simulink model "Blupanda"  (R2023a)
settings: Solver=VariableStepAuto  StartTime=0.0  StopTime=10.0  RelTol=1e-3
(part 2 of 2)

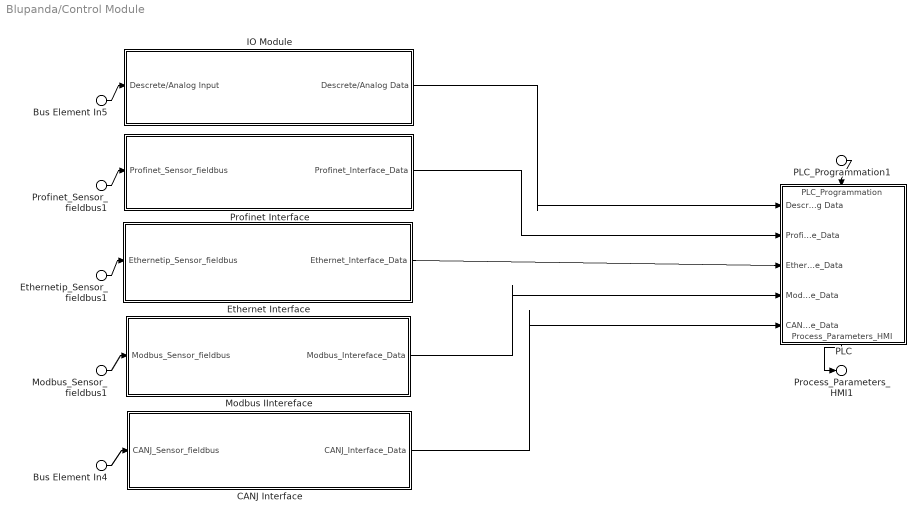
== system Blupanda/Control Module ==
  PLC_Programmation1 : Inport  PortName=PLC_Programmation
  Profinet_Sensor_fieldbus1 : Inport  Port=2  PortName=Profinet_Sensor_fieldbus
  Ethernetip_Sensor_fieldbus1 : Inport  Port=3  PortName=Ethernetip_Sensor_fieldbus
  Bus Element In4 : Inport  Port=4  PortName=CANJ_Sensor_fieldbus
  Bus Element In5 : Inport  Port=5  PortName=Descrete/Analog Input
  Modbus_Sensor_fieldbus1 : Inport  Port=6  PortName=Modbus_Sensor_fieldbus
  CANJ Interface : Subsystem
      settings: PortSchema="{\"entries\":[{\"content\":{\"headerSize\":26,\"margin\":15,\"minimumSpacing\":25,\"sides\":[{\"content\":{\"connectorIds\":[\"In1\"]},\"type\":\"ConnectorPlacement.EquallySpacedRectSide\",\"uuid\":\"ff8f3bf2-d6f6-4ecc-9677-a0e5f5ade440\"},{\"content\":{\"connectorIds\":[\"Out1\"],\"side\":\"RIGHT\"},\"type\":\"ConnectorPlacement.EquallySpacedRectSide\",\"uuid\":\"fe155757-f3d5-40d8-a583-dbbc24843437\"},{\"content\":{\"side\":\"TOP\"},\"type\":\"ConnectorPlacement.EquallySpacedRectSide\",\"uuid\":\"51bc4fd0-0675-45de-93bd-0dc8d94c5489\"}]},\"type\":\"ConnectorPlacement.EquallySpacedConnector\",\"uuid\":\"7eb8fdf8-dbe2-49f3-b9bd-384f85dcc997\"}],\"packageUris\":[\"http://schema.mathworks.com/mf0/Connector/R2020b\"],\"version\":\"1.0\"}"
  Ethernet Interface : Subsystem
      settings: PortSchema="{\"entries\":[{\"content\":{\"headerSize\":26,\"margin\":15,\"minimumSpacing\":25,\"sides\":[{\"content\":{\"connectorIds\":[\"In1\"]},\"type\":\"ConnectorPlacement.EquallySpacedRectSide\",\"uuid\":\"ff8f3bf2-d6f6-4ecc-9677-a0e5f5ade440\"},{\"content\":{\"connectorIds\":[\"Out1\"],\"side\":\"RIGHT\"},\"type\":\"ConnectorPlacement.EquallySpacedRectSide\",\"uuid\":\"fe155757-f3d5-40d8-a583-dbbc24843437\"},{\"content\":{\"side\":\"TOP\"},\"type\":\"ConnectorPlacement.EquallySpacedRectSide\",\"uuid\":\"51bc4fd0-0675-45de-93bd-0dc8d94c5489\"}]},\"type\":\"ConnectorPlacement.EquallySpacedConnector\",\"uuid\":\"7eb8fdf8-dbe2-49f3-b9bd-384f85dcc997\"}],\"packageUris\":[\"http://schema.mathworks.com/mf0/Connector/R2020b\"],\"version\":\"1.0\"}"
  IO Module : Subsystem
      settings: PortSchema="{\"entries\":[{\"content\":{\"headerSize\":26,\"margin\":15,\"minimumSpacing\":25,\"sides\":[{\"content\":{\"connectorIds\":[\"In1\"]},\"type\":\"ConnectorPlacement.EquallySpacedRectSide\",\"uuid\":\"ff8f3bf2-d6f6-4ecc-9677-a0e5f5ade440\"},{\"content\":{\"connectorIds\":[\"Out1\"],\"side\":\"RIGHT\"},\"type\":\"ConnectorPlacement.EquallySpacedRectSide\",\"uuid\":\"fe155757-f3d5-40d8-a583-dbbc24843437\"},{\"content\":{\"side\":\"TOP\"},\"type\":\"ConnectorPlacement.EquallySpacedRectSide\",\"uuid\":\"51bc4fd0-0675-45de-93bd-0dc8d94c5489\"}]},\"type\":\"ConnectorPlacement.EquallySpacedConnector\",\"uuid\":\"7eb8fdf8-dbe2-49f3-b9bd-384f85dcc997\"}],\"packageUris\":[\"http://schema.mathworks.com/mf0/Connector/R2020b\"],\"version\":\"1.0\"}"
  Modbus IIntereface : Subsystem
      settings: PortSchema="{\"entries\":[{\"content\":{\"headerSize\":26,\"margin\":15,\"minimumSpacing\":25,\"sides\":[{\"content\":{\"connectorIds\":[\"In1\"]},\"type\":\"ConnectorPlacement.EquallySpacedRectSide\",\"uuid\":\"ff8f3bf2-d6f6-4ecc-9677-a0e5f5ade440\"},{\"content\":{\"connectorIds\":[\"Out1\"],\"side\":\"RIGHT\"},\"type\":\"ConnectorPlacement.EquallySpacedRectSide\",\"uuid\":\"fe155757-f3d5-40d8-a583-dbbc24843437\"},{\"content\":{\"side\":\"TOP\"},\"type\":\"ConnectorPlacement.EquallySpacedRectSide\",\"uuid\":\"51bc4fd0-0675-45de-93bd-0dc8d94c5489\"}]},\"type\":\"ConnectorPlacement.EquallySpacedConnector\",\"uuid\":\"7eb8fdf8-dbe2-49f3-b9bd-384f85dcc997\"}],\"packageUris\":[\"http://schema.mathworks.com/mf0/Connector/R2020b\"],\"version\":\"1.0\"}"
  PLC : Subsystem
      settings: PortSchema="{\"entries\":[{\"content\":{\"headerSize\":26,\"margin\":15,\"minimumSpacing\":25,\"sides\":[{\"content\":{\"connectorIds\":[\"In1\",\"In4\",\"In5\",\"In6\",\"In2\"]},\"type\":\"ConnectorPlacement.EquallySpacedRectSide\",\"uuid\":\"ff8f3bf2-d6f6-4ecc-9677-a0e5f5ade440\"},{\"content\":{\"side\":\"RIGHT\"},\"type\":\"ConnectorPlacement.EquallySpacedRectSide\",\"uuid\":\"fe155757-f3d5-40d8-a583-dbbc24843437\"},{\"content\":{\"connectorIds\":[\"In3\"],\"side\":\"TOP\"},\"type\":\"ConnectorPlacement.EquallySpacedRectSide\",\"uuid\":\"51bc4fd0-0675-45de-93bd-0dc8d94c5489\"},{\"content\":{\"connectorIds\":[\"Out1\"],\"side\":\"BOTTOM\"},\"type\":\"ConnectorPlacement.EquallySpacedRectSide\",\"uuid\":\"b7b44f41-0e2c-4bbd-9aa1-2b70573de7d3\"}]},\"type\":\"ConnectorPlacement.EquallySpacedConnector\",\"uuid\":\"7eb8fdf8-dbe2-49f3-b9bd-384f85dcc997\"}],\"packageUris\":[\"http://schema.mathworks.com/mf0/Connector/R2020b\"],\"version\":\"1.0\"}"
  Profinet Interface : Subsystem
      settings: PortSchema="{\"entries\":[{\"content\":{\"headerSize\":26,\"margin\":15,\"minimumSpacing\":25,\"sides\":[{\"content\":{\"connectorIds\":[\"In1\"]},\"type\":\"ConnectorPlacement.EquallySpacedRectSide\",\"uuid\":\"ff8f3bf2-d6f6-4ecc-9677-a0e5f5ade440\"},{\"content\":{\"connectorIds\":[\"Out1\"],\"side\":\"RIGHT\"},\"type\":\"ConnectorPlacement.EquallySpacedRectSide\",\"uuid\":\"fe155757-f3d5-40d8-a583-dbbc24843437\"},{\"content\":{\"side\":\"TOP\"},\"type\":\"ConnectorPlacement.EquallySpacedRectSide\",\"uuid\":\"51bc4fd0-0675-45de-93bd-0dc8d94c5489\"}]},\"type\":\"ConnectorPlacement.EquallySpacedConnector\",\"uuid\":\"7eb8fdf8-dbe2-49f3-b9bd-384f85dcc997\"}],\"packageUris\":[\"http://schema.mathworks.com/mf0/Connector/R2020b\"],\"version\":\"1.0\"}"
  Process_Parameters_HMI1 : Outport  PortName=Process_Parameters_HMI
  wires:
  Modbus_Sensor_fieldbus1/1 -> Modbus IIntereface/1(Modbus_Sensor_fieldbus)
  Profinet_Sensor_fieldbus1/1 -> Profinet Interface/1(Profinet_Sensor_fieldbus)
  Ethernetip_Sensor_fieldbus1/1 -> Ethernet Interface/1(Ethernetip_Sensor_fieldbus)
  Profinet Interface/1(Profinet_Interface_Data) -> PLC/4(Profinet_Interface_Data)
  Modbus IIntereface/1(Modbus_Intereface_Data) -> PLC/6(Modbus_Intereface_Data)
  PLC/1(Process_Parameters_HMI) -> Process_Parameters_HMI1/1
  Ethernet Interface/1(Ethernet_Interface_Data) -> PLC/5(Ethernet_Interface_Data)
  PLC_Programmation1/1 -> PLC/3(PLC_Programmation)
  CANJ Interface/1(CANJ_Interface_Data) -> PLC/2(CANJ_Interface_Data)
  Bus Element In4/1 -> CANJ Interface/1(CANJ_Sensor_fieldbus)
  IO Module/1(Descrete/Analog Data) -> PLC/1(Descrete/Analog Data)
  Bus Element In5/1 -> IO Module/1(Descrete/Analog Input)

== system Blupanda/Deutsch 6-pin Connector ==
  Bus Element In1 : Inport  PortName=XGCS460B201_CANJ_Data
  Bus Element Out1 : Outport  PortName=CANJ_Sensor_fieldbus

== system Blupanda/EthernetIP_network ==
  Bus Element In1 : Inport  PortName=ethernet ip data
  Bus Element Out1 : Outport  PortName=Ethernetip_Sensor_fieldbus

== system Blupanda/HMI ==
  Bus Element In1 : Inport  PortName=Process_Parameters_HMI

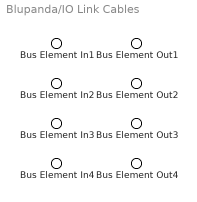
== system Blupanda/IO Link Cables ==
  Bus Element In1 : Inport  PortName=XGCS 89 01201_IOLimk_data
  Bus Element In2 : Inport  Port=2  PortName=XGCS 49 01201_IOLink_data
  Bus Element In3 : Inport  Port=3  PortName=M18_IOLink_data
  Bus Element In4 : Inport  Port=4  PortName=M30_IOLink_data
  Bus Element Out1 : Outport  PortName=XGCS 89 01201_IOLimk_data_2_master
  Bus Element Out2 : Outport  Port=2  PortName=XGCS 49 01201_IOLink_data_2_master
  Bus Element Out3 : Outport  Port=3  PortName=M18_IOLink_data_2_master
  Bus Element Out4 : Outport  Port=4  PortName=M30_IOLink_data_2_masters

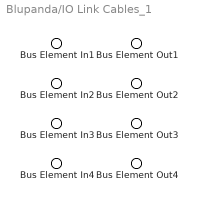
== system Blupanda/IO Link Cables_1 ==
  Bus Element In1 : Inport  PortName=XGCS 89 01201_IOLimk_data
  Bus Element In2 : Inport  Port=2  PortName=XGCS 49 01201_IOLink_data
  Bus Element In3 : Inport  Port=3  PortName=M18_IOLink_data
  Bus Element In4 : Inport  Port=4  PortName=M30_IOLink_data
  Bus Element Out1 : Outport  PortName=XGCS 89 01201_IOLimk_data_2_master
  Bus Element Out2 : Outport  Port=2  PortName=XGCS 49 01201_IOLink_data_2_master
  Bus Element Out3 : Outport  Port=3  PortName=M18_IOLink_data_2_master
  Bus Element Out4 : Outport  Port=4  PortName=M30_IOLink_data_2_masters

== system Blupanda/IOLink_master_EthernetIP ==
  Bus Element In1 : Inport  PortName=XGCS 49 01201_IOLink_data
  Bus Element In2 : Inport  Port=2  PortName=XGCS 89 01201_IOLimk_data
  Bus Element In3 : Inport  Port=3  PortName=M18_IOLink_data
  Bus Element In4 : Inport  Port=4  PortName=M30_IOLink_data
  Bus Element Out1 : Outport  PortName=IOLink_master_Profinet_serial_data_EthernetIP

== system Blupanda/IOLink_master_Profinet ==
  Bus Element In1 : Inport  PortName=XGCS 89 01201_IOLimk_data_2_master
  Bus Element In2 : Inport  Port=2  PortName=XGCS 49 01201_IOLink_data_2_master
  Bus Element In3 : Inport  Port=3  PortName=M18_IOLink_data_2_master
  Bus Element In4 : Inport  Port=4  PortName=M30_IOLink_data_2_masters
  Bus Element Out1 : Outport  PortName=IOLink_master_Profinet_serial_data_profinet

== system Blupanda/Interface_box_network_1 ==
  Bus Element In1 : Inport  PortName="XGSZ84 PNT  _serial_data_Profinet"
  Bus Element Out1 : Outport  PortName="XGSZ84 PNT  _serial_data_Profinet_2_network"

== system Blupanda/Interface_box_network_2 ==
  Bus Element In1 : Inport  PortName=XGSZ 84 EIP _serial_data_ethernet
  Bus Element Out1 : Outport  PortName=XGSZ 84 EIP _serial_data_ethernet_2_network

== system Blupanda/Interface_box_network_3 ==
  Bus Element In1 : Inport  PortName=XGSZ84 ETH _serial_data_Mobdus
  Bus Element Out1 : Outport  PortName=XGSZ84 ETH _serial_data_Mobdus_2_network

== system Blupanda/M12 to Ethernet 0 ==
  Bus Element In1 : Inport  PortName=XGCS 850C 201_ModusTCp_Data
  Bus Element Out1 : Outport  PortName=""

== system Blupanda/M12 to Ethernet 1 ==
  Bus Element In1 : Inport  PortName=XGCS 850C 201_Ethernetp_Data
  Bus Element Out1 : Outport  PortName=XGCS 850C 201_Ethernetp_Data_2_swtich

== system Blupanda/M12 to Ethernet 2 ==
  Bus Element In1 : Inport  PortName=XGCS 850C 201_Profinet_Data
  Bus Element Out1 : Outport  PortName=XGCS 850C 201_Profinet_Data_2_network

== system Blupanda/ModbusTCP_Network ==
  Bus Element In1 : Inport  PortName=XGSZ84 ETH _serial_data_Mobdus_2_network
  Bus Element In2 : Inport  Port=2  PortName=XGCS 850C 201_ModusTCp_Data_2_network
  Bus Element Out1 : Outport  PortName=Modbus_Sensor_fieldbus

== system Blupanda/Profinet_network ==
  Bus Element In2 : Inport  PortName=IOLink_master_Profinet_serial_data_profinet
  Bus Element In1 : Inport  Port=2  PortName="XGSZ84 PNT  _serial_data_Profinet_2_network"
  Bus Element In3 : Inport  Port=3  PortName=XGCS 850C 201_Profinet_Data
  Bus Element Out1 : Outport  PortName=Profinet_Sensor_fieldbus

== system Blupanda/RFID_CANJ ==
  XGCS460B201 : Subsystem
      settings: PortSchema="{\"entries\":[{\"content\":{\"headerSize\":26,\"margin\":15,\"minimumSpacing\":25,\"sides\":[{\"content\":{},\"type\":\"ConnectorPlacement.EquallySpacedRectSide\",\"uuid\":\"ff8f3bf2-d6f6-4ecc-9677-a0e5f5ade440\"},{\"content\":{\"connectorIds\":[\"Out1\"],\"side\":\"RIGHT\"},\"type\":\"ConnectorPlacement.EquallySpacedRectSide\",\"uuid\":\"fe155757-f3d5-40d8-a583-dbbc24843437\"},{\"content\":{\"side\":\"TOP\"},\"type\":\"ConnectorPlacement.EquallySpacedRectSide\",\"uuid\":\"51bc4fd0-0675-45de-93bd-0dc8d94c5489\"}]},\"type\":\"ConnectorPlacement.EquallySpacedConnector\",\"uuid\":\"7eb8fdf8-dbe2-49f3-b9bd-384f85dcc997\"}],\"packageUris\":[\"http://schema.mathworks.com/mf0/Connector/R2020b\"],\"version\":\"1.0\"}"
  XGCS460B202_CANJ_Data1 : Outport  PortName=XGCS460B201_CANJ_Data
  wires:
  XGCS460B201/1(XGCS460B201_CANJ_Data) -> XGCS460B202_CANJ_Data1/1

== system Blupanda/RFID_EthernetIP ==
  "XGCS 850C 201 " : Subsystem
      settings: PortSchema="{\"entries\":[{\"content\":{\"headerSize\":26,\"margin\":15,\"minimumSpacing\":25,\"sides\":[{\"content\":{},\"type\":\"ConnectorPlacement.EquallySpacedRectSide\",\"uuid\":\"ff8f3bf2-d6f6-4ecc-9677-a0e5f5ade440\"},{\"content\":{\"side\":\"RIGHT\"},\"type\":\"ConnectorPlacement.EquallySpacedRectSide\",\"uuid\":\"fe155757-f3d5-40d8-a583-dbbc24843437\"},{\"content\":{\"connectorIds\":[\"Out1\"],\"side\":\"TOP\"},\"type\":\"ConnectorPlacement.EquallySpacedRectSide\",\"uuid\":\"51bc4fd0-0675-45de-93bd-0dc8d94c5489\"},{\"content\":{\"side\":\"BOTTOM\"},\"type\":\"ConnectorPlacement.EquallySpacedRectSide\",\"uuid\":\"69d4bc1c-5af7-467d-9dcb-7dfd5dc85590\"}]},\"type\":\"ConnectorPlacement.EquallySpacedConnector\",\"uuid\":\"7eb8fdf8-dbe2-49f3-b9bd-384f85dcc997\"}],\"packageUris\":[\"http://schema.mathworks.com/mf0/Connector/R2020b\"],\"version\":\"1.0\"}"
  XGCS 850C 201_Ethernetp_Data1 : Outport  PortName=XGCS 850C 201_Ethernetp_Data
  wires:
  "XGCS 850C 201 "/1(XGCS 850C 201_Ethernetp_Data) -> XGCS 850C 201_Ethernetp_Data1/1

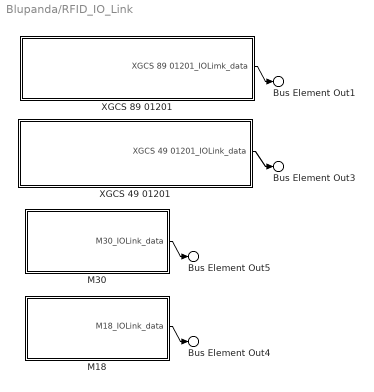
== system Blupanda/RFID_IO_Link ==
  M18 : Subsystem
      settings: PortSchema="{\"entries\":[{\"content\":{\"headerSize\":26,\"margin\":15,\"minimumSpacing\":25,\"sides\":[{\"content\":{},\"type\":\"ConnectorPlacement.EquallySpacedRectSide\",\"uuid\":\"ff8f3bf2-d6f6-4ecc-9677-a0e5f5ade440\"},{\"content\":{\"connectorIds\":[\"Out1\"],\"side\":\"RIGHT\"},\"type\":\"ConnectorPlacement.EquallySpacedRectSide\",\"uuid\":\"fe155757-f3d5-40d8-a583-dbbc24843437\"},{\"content\":{\"side\":\"TOP\"},\"type\":\"ConnectorPlacement.EquallySpacedRectSide\",\"uuid\":\"51bc4fd0-0675-45de-93bd-0dc8d94c5489\"}]},\"type\":\"ConnectorPlacement.EquallySpacedConnector\",\"uuid\":\"7eb8fdf8-dbe2-49f3-b9bd-384f85dcc997\"}],\"packageUris\":[\"http://schema.mathworks.com/mf0/Connector/R2020b\"],\"version\":\"1.0\"}"
  M30 : Subsystem
      settings: PortSchema="{\"entries\":[{\"content\":{\"headerSize\":26,\"margin\":15,\"minimumSpacing\":25,\"sides\":[{\"content\":{},\"type\":\"ConnectorPlacement.EquallySpacedRectSide\",\"uuid\":\"ff8f3bf2-d6f6-4ecc-9677-a0e5f5ade440\"},{\"content\":{\"connectorIds\":[\"Out1\"],\"side\":\"RIGHT\"},\"type\":\"ConnectorPlacement.EquallySpacedRectSide\",\"uuid\":\"fe155757-f3d5-40d8-a583-dbbc24843437\"},{\"content\":{\"side\":\"TOP\"},\"type\":\"ConnectorPlacement.EquallySpacedRectSide\",\"uuid\":\"51bc4fd0-0675-45de-93bd-0dc8d94c5489\"}]},\"type\":\"ConnectorPlacement.EquallySpacedConnector\",\"uuid\":\"7eb8fdf8-dbe2-49f3-b9bd-384f85dcc997\"}],\"packageUris\":[\"http://schema.mathworks.com/mf0/Connector/R2020b\"],\"version\":\"1.0\"}"
  XGCS 49 01201 : Subsystem
      settings: PortSchema="{\"entries\":[{\"content\":{\"headerSize\":26,\"margin\":15,\"minimumSpacing\":25,\"sides\":[{\"content\":{},\"type\":\"ConnectorPlacement.EquallySpacedRectSide\",\"uuid\":\"ff8f3bf2-d6f6-4ecc-9677-a0e5f5ade440\"},{\"content\":{\"connectorIds\":[\"Out1\"],\"side\":\"RIGHT\"},\"type\":\"ConnectorPlacement.EquallySpacedRectSide\",\"uuid\":\"fe155757-f3d5-40d8-a583-dbbc24843437\"},{\"content\":{\"side\":\"TOP\"},\"type\":\"ConnectorPlacement.EquallySpacedRectSide\",\"uuid\":\"51bc4fd0-0675-45de-93bd-0dc8d94c5489\"}]},\"type\":\"ConnectorPlacement.EquallySpacedConnector\",\"uuid\":\"7eb8fdf8-dbe2-49f3-b9bd-384f85dcc997\"}],\"packageUris\":[\"http://schema.mathworks.com/mf0/Connector/R2020b\"],\"version\":\"1.0\"}"
  XGCS 89 01201 : Subsystem
      settings: PortSchema="{\"entries\":[{\"content\":{\"headerSize\":26,\"margin\":15,\"minimumSpacing\":25,\"sides\":[{\"content\":{},\"type\":\"ConnectorPlacement.EquallySpacedRectSide\",\"uuid\":\"ff8f3bf2-d6f6-4ecc-9677-a0e5f5ade440\"},{\"content\":{\"connectorIds\":[\"Out1\"],\"side\":\"RIGHT\"},\"type\":\"ConnectorPlacement.EquallySpacedRectSide\",\"uuid\":\"fe155757-f3d5-40d8-a583-dbbc24843437\"},{\"content\":{\"side\":\"TOP\"},\"type\":\"ConnectorPlacement.EquallySpacedRectSide\",\"uuid\":\"51bc4fd0-0675-45de-93bd-0dc8d94c5489\"}]},\"type\":\"ConnectorPlacement.EquallySpacedConnector\",\"uuid\":\"7eb8fdf8-dbe2-49f3-b9bd-384f85dcc997\"}],\"packageUris\":[\"http://schema.mathworks.com/mf0/Connector/R2020b\"],\"version\":\"1.0\"}"
  Bus Element Out1 : Outport  PortName=XGCS 89 01201_IOLimk_data
  Bus Element Out3 : Outport  Port=2  PortName=XGCS 49 01201_IOLink_data
  Bus Element Out4 : Outport  Port=3  PortName=M18_IOLink_data
  Bus Element Out5 : Outport  Port=4  PortName=M30_IOLink_data
  wires:
  XGCS 89 01201/1(XGCS 89 01201_IOLimk_data) -> Bus Element Out1/1
  XGCS 49 01201/1(XGCS 49 01201_IOLink_data) -> Bus Element Out3/1
  M30/1(M30_IOLink_data) -> Bus Element Out5/1
  M18/1(M18_IOLink_data) -> Bus Element Out4/1

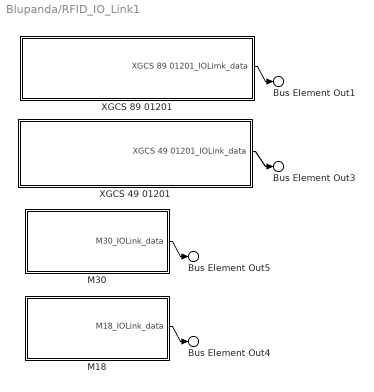
== system Blupanda/RFID_IO_Link1 ==
  M18 : Subsystem
      settings: PortSchema="{\"entries\":[{\"content\":{\"headerSize\":26,\"margin\":15,\"minimumSpacing\":25,\"sides\":[{\"content\":{},\"type\":\"ConnectorPlacement.EquallySpacedRectSide\",\"uuid\":\"ff8f3bf2-d6f6-4ecc-9677-a0e5f5ade440\"},{\"content\":{\"connectorIds\":[\"Out1\"],\"side\":\"RIGHT\"},\"type\":\"ConnectorPlacement.EquallySpacedRectSide\",\"uuid\":\"fe155757-f3d5-40d8-a583-dbbc24843437\"},{\"content\":{\"side\":\"TOP\"},\"type\":\"ConnectorPlacement.EquallySpacedRectSide\",\"uuid\":\"51bc4fd0-0675-45de-93bd-0dc8d94c5489\"}]},\"type\":\"ConnectorPlacement.EquallySpacedConnector\",\"uuid\":\"7eb8fdf8-dbe2-49f3-b9bd-384f85dcc997\"}],\"packageUris\":[\"http://schema.mathworks.com/mf0/Connector/R2020b\"],\"version\":\"1.0\"}"
  M30 : Subsystem
      settings: PortSchema="{\"entries\":[{\"content\":{\"headerSize\":26,\"margin\":15,\"minimumSpacing\":25,\"sides\":[{\"content\":{},\"type\":\"ConnectorPlacement.EquallySpacedRectSide\",\"uuid\":\"ff8f3bf2-d6f6-4ecc-9677-a0e5f5ade440\"},{\"content\":{\"connectorIds\":[\"Out1\"],\"side\":\"RIGHT\"},\"type\":\"ConnectorPlacement.EquallySpacedRectSide\",\"uuid\":\"fe155757-f3d5-40d8-a583-dbbc24843437\"},{\"content\":{\"side\":\"TOP\"},\"type\":\"ConnectorPlacement.EquallySpacedRectSide\",\"uuid\":\"51bc4fd0-0675-45de-93bd-0dc8d94c5489\"}]},\"type\":\"ConnectorPlacement.EquallySpacedConnector\",\"uuid\":\"7eb8fdf8-dbe2-49f3-b9bd-384f85dcc997\"}],\"packageUris\":[\"http://schema.mathworks.com/mf0/Connector/R2020b\"],\"version\":\"1.0\"}"
  XGCS 49 01201 : Subsystem
      settings: PortSchema="{\"entries\":[{\"content\":{\"headerSize\":26,\"margin\":15,\"minimumSpacing\":25,\"sides\":[{\"content\":{},\"type\":\"ConnectorPlacement.EquallySpacedRectSide\",\"uuid\":\"ff8f3bf2-d6f6-4ecc-9677-a0e5f5ade440\"},{\"content\":{\"connectorIds\":[\"Out1\"],\"side\":\"RIGHT\"},\"type\":\"ConnectorPlacement.EquallySpacedRectSide\",\"uuid\":\"fe155757-f3d5-40d8-a583-dbbc24843437\"},{\"content\":{\"side\":\"TOP\"},\"type\":\"ConnectorPlacement.EquallySpacedRectSide\",\"uuid\":\"51bc4fd0-0675-45de-93bd-0dc8d94c5489\"}]},\"type\":\"ConnectorPlacement.EquallySpacedConnector\",\"uuid\":\"7eb8fdf8-dbe2-49f3-b9bd-384f85dcc997\"}],\"packageUris\":[\"http://schema.mathworks.com/mf0/Connector/R2020b\"],\"version\":\"1.0\"}"
  XGCS 89 01201 : Subsystem
      settings: PortSchema="{\"entries\":[{\"content\":{\"headerSize\":26,\"margin\":15,\"minimumSpacing\":25,\"sides\":[{\"content\":{},\"type\":\"ConnectorPlacement.EquallySpacedRectSide\",\"uuid\":\"ff8f3bf2-d6f6-4ecc-9677-a0e5f5ade440\"},{\"content\":{\"connectorIds\":[\"Out1\"],\"side\":\"RIGHT\"},\"type\":\"ConnectorPlacement.EquallySpacedRectSide\",\"uuid\":\"fe155757-f3d5-40d8-a583-dbbc24843437\"},{\"content\":{\"side\":\"TOP\"},\"type\":\"ConnectorPlacement.EquallySpacedRectSide\",\"uuid\":\"51bc4fd0-0675-45de-93bd-0dc8d94c5489\"}]},\"type\":\"ConnectorPlacement.EquallySpacedConnector\",\"uuid\":\"7eb8fdf8-dbe2-49f3-b9bd-384f85dcc997\"}],\"packageUris\":[\"http://schema.mathworks.com/mf0/Connector/R2020b\"],\"version\":\"1.0\"}"
  Bus Element Out1 : Outport  PortName=XGCS 89 01201_IOLimk_data
  Bus Element Out3 : Outport  Port=2  PortName=XGCS 49 01201_IOLink_data
  Bus Element Out4 : Outport  Port=3  PortName=M18_IOLink_data
  Bus Element Out5 : Outport  Port=4  PortName=M30_IOLink_data
  wires:
  XGCS 89 01201/1(XGCS 89 01201_IOLimk_data) -> Bus Element Out1/1
  XGCS 49 01201/1(XGCS 49 01201_IOLink_data) -> Bus Element Out3/1
  M30/1(M30_IOLink_data) -> Bus Element Out5/1
  M18/1(M18_IOLink_data) -> Bus Element Out4/1

== system Blupanda/RFID_Modbus ==
  XGCS 850C 201 : Subsystem
      settings: PortSchema="{\"entries\":[{\"content\":{\"headerSize\":26,\"margin\":15,\"minimumSpacing\":25,\"sides\":[{\"content\":{},\"type\":\"ConnectorPlacement.EquallySpacedRectSide\",\"uuid\":\"ff8f3bf2-d6f6-4ecc-9677-a0e5f5ade440\"},{\"content\":{\"side\":\"RIGHT\"},\"type\":\"ConnectorPlacement.EquallySpacedRectSide\",\"uuid\":\"fe155757-f3d5-40d8-a583-dbbc24843437\"},{\"content\":{\"connectorIds\":[\"Out1\"],\"side\":\"TOP\"},\"type\":\"ConnectorPlacement.EquallySpacedRectSide\",\"uuid\":\"51bc4fd0-0675-45de-93bd-0dc8d94c5489\"}]},\"type\":\"ConnectorPlacement.EquallySpacedConnector\",\"uuid\":\"7eb8fdf8-dbe2-49f3-b9bd-384f85dcc997\"}],\"packageUris\":[\"http://schema.mathworks.com/mf0/Connector/R2020b\"],\"version\":\"1.0\"}"
  XGCS 850C 201_ModusTCp_Data1 : Outport  PortName=XGCS 850C 201_ModusTCp_Data
  wires:
  XGCS 850C 201/1(XGCS 850C 201_ModusTCp_Data) -> XGCS 850C 201_ModusTCp_Data1/1

== system Blupanda/RFID_PNP ==
  "XGCS49 1 B201 " : Subsystem
      settings: PortSchema="{\"entries\":[{\"content\":{\"headerSize\":26,\"margin\":15,\"minimumSpacing\":25,\"sides\":[{\"content\":{},\"type\":\"ConnectorPlacement.EquallySpacedRectSide\",\"uuid\":\"ff8f3bf2-d6f6-4ecc-9677-a0e5f5ade440\"},{\"content\":{\"connectorIds\":[\"Out1\"],\"side\":\"RIGHT\"},\"type\":\"ConnectorPlacement.EquallySpacedRectSide\",\"uuid\":\"fe155757-f3d5-40d8-a583-dbbc24843437\"},{\"content\":{\"connectorIds\":[\"In1\",\"In2\"],\"side\":\"TOP\"},\"type\":\"ConnectorPlacement.EquallySpacedRectSide\",\"uuid\":\"51bc4fd0-0675-45de-93bd-0dc8d94c5489\"}]},\"type\":\"ConnectorPlacement.EquallySpacedConnector\",\"uuid\":\"7eb8fdf8-dbe2-49f3-b9bd-384f85dcc997\"}],\"packageUris\":[\"http://schema.mathworks.com/mf0/Connector/R2020b\"],\"version\":\"1.0\"}"
  XGCS49 1 B201_PNP_Data1 : Outport  PortName=XGCS49 1 B201_PNP_Data
  wires:
  "XGCS49 1 B201 "/1(XGCS49 1 B201_PNP_Data) -> XGCS49 1 B201_PNP_Data1/1

== system Blupanda/RFID_Profinet ==
  "XGCS 850C 201 " : Subsystem
      settings: PortSchema="{\"entries\":[{\"content\":{\"headerSize\":26,\"margin\":15,\"minimumSpacing\":25,\"sides\":[{\"content\":{},\"type\":\"ConnectorPlacement.EquallySpacedRectSide\",\"uuid\":\"ff8f3bf2-d6f6-4ecc-9677-a0e5f5ade440\"},{\"content\":{\"side\":\"RIGHT\"},\"type\":\"ConnectorPlacement.EquallySpacedRectSide\",\"uuid\":\"fe155757-f3d5-40d8-a583-dbbc24843437\"},{\"content\":{\"connectorIds\":[\"Out1\"],\"side\":\"TOP\"},\"type\":\"ConnectorPlacement.EquallySpacedRectSide\",\"uuid\":\"51bc4fd0-0675-45de-93bd-0dc8d94c5489\"}]},\"type\":\"ConnectorPlacement.EquallySpacedConnector\",\"uuid\":\"7eb8fdf8-dbe2-49f3-b9bd-384f85dcc997\"}],\"packageUris\":[\"http://schema.mathworks.com/mf0/Connector/R2020b\"],\"version\":\"1.0\"}"
  Bus Element Out1 : Outport  PortName=XGCS 850C 201_Profinet_Data
  wires:
  "XGCS 850C 201 "/1(XGCS 850C 201_Profinet_Data) -> Bus Element Out1/1

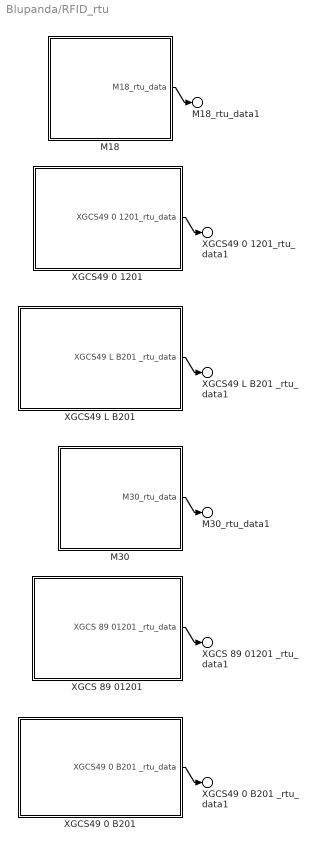
== system Blupanda/RFID_rtu ==
  M18 : Subsystem
      settings: PortSchema="{\"entries\":[{\"content\":{\"headerSize\":26,\"margin\":15,\"minimumSpacing\":25,\"sides\":[{\"content\":{},\"type\":\"ConnectorPlacement.EquallySpacedRectSide\",\"uuid\":\"ff8f3bf2-d6f6-4ecc-9677-a0e5f5ade440\"},{\"content\":{\"connectorIds\":[\"Out1\"],\"side\":\"RIGHT\"},\"type\":\"ConnectorPlacement.EquallySpacedRectSide\",\"uuid\":\"fe155757-f3d5-40d8-a583-dbbc24843437\"},{\"content\":{\"side\":\"TOP\"},\"type\":\"ConnectorPlacement.EquallySpacedRectSide\",\"uuid\":\"51bc4fd0-0675-45de-93bd-0dc8d94c5489\"}]},\"type\":\"ConnectorPlacement.EquallySpacedConnector\",\"uuid\":\"7eb8fdf8-dbe2-49f3-b9bd-384f85dcc997\"}],\"packageUris\":[\"http://schema.mathworks.com/mf0/Connector/R2020b\"],\"version\":\"1.0\"}"
  M30 : Subsystem
      settings: PortSchema="{\"entries\":[{\"content\":{\"headerSize\":26,\"margin\":15,\"minimumSpacing\":25,\"sides\":[{\"content\":{},\"type\":\"ConnectorPlacement.EquallySpacedRectSide\",\"uuid\":\"ff8f3bf2-d6f6-4ecc-9677-a0e5f5ade440\"},{\"content\":{\"connectorIds\":[\"Out1\"],\"side\":\"RIGHT\"},\"type\":\"ConnectorPlacement.EquallySpacedRectSide\",\"uuid\":\"fe155757-f3d5-40d8-a583-dbbc24843437\"},{\"content\":{\"side\":\"TOP\"},\"type\":\"ConnectorPlacement.EquallySpacedRectSide\",\"uuid\":\"51bc4fd0-0675-45de-93bd-0dc8d94c5489\"}]},\"type\":\"ConnectorPlacement.EquallySpacedConnector\",\"uuid\":\"7eb8fdf8-dbe2-49f3-b9bd-384f85dcc997\"}],\"packageUris\":[\"http://schema.mathworks.com/mf0/Connector/R2020b\"],\"version\":\"1.0\"}"
  "XGCS 89 01201 " : Subsystem
      settings: PortSchema="{\"entries\":[{\"content\":{\"headerSize\":26,\"margin\":15,\"minimumSpacing\":25,\"sides\":[{\"content\":{},\"type\":\"ConnectorPlacement.EquallySpacedRectSide\",\"uuid\":\"ff8f3bf2-d6f6-4ecc-9677-a0e5f5ade440\"},{\"content\":{\"connectorIds\":[\"Out1\"],\"side\":\"RIGHT\"},\"type\":\"ConnectorPlacement.EquallySpacedRectSide\",\"uuid\":\"fe155757-f3d5-40d8-a583-dbbc24843437\"},{\"content\":{\"side\":\"TOP\"},\"type\":\"ConnectorPlacement.EquallySpacedRectSide\",\"uuid\":\"51bc4fd0-0675-45de-93bd-0dc8d94c5489\"}]},\"type\":\"ConnectorPlacement.EquallySpacedConnector\",\"uuid\":\"7eb8fdf8-dbe2-49f3-b9bd-384f85dcc997\"}],\"packageUris\":[\"http://schema.mathworks.com/mf0/Connector/R2020b\"],\"version\":\"1.0\"}"
  "XGCS49 0 1201 " : Subsystem
      settings: PortSchema="{\"entries\":[{\"content\":{\"headerSize\":26,\"margin\":15,\"minimumSpacing\":25,\"sides\":[{\"content\":{},\"type\":\"ConnectorPlacement.EquallySpacedRectSide\",\"uuid\":\"ff8f3bf2-d6f6-4ecc-9677-a0e5f5ade440\"},{\"content\":{\"connectorIds\":[\"Out1\"],\"side\":\"RIGHT\"},\"type\":\"ConnectorPlacement.EquallySpacedRectSide\",\"uuid\":\"fe155757-f3d5-40d8-a583-dbbc24843437\"},{\"content\":{\"side\":\"TOP\"},\"type\":\"ConnectorPlacement.EquallySpacedRectSide\",\"uuid\":\"51bc4fd0-0675-45de-93bd-0dc8d94c5489\"}]},\"type\":\"ConnectorPlacement.EquallySpacedConnector\",\"uuid\":\"7eb8fdf8-dbe2-49f3-b9bd-384f85dcc997\"}],\"packageUris\":[\"http://schema.mathworks.com/mf0/Connector/R2020b\"],\"version\":\"1.0\"}"
  "XGCS49 0 B201 " : Subsystem
      settings: PortSchema="{\"entries\":[{\"content\":{\"headerSize\":26,\"margin\":15,\"minimumSpacing\":25,\"sides\":[{\"content\":{},\"type\":\"ConnectorPlacement.EquallySpacedRectSide\",\"uuid\":\"ff8f3bf2-d6f6-4ecc-9677-a0e5f5ade440\"},{\"content\":{\"connectorIds\":[\"Out1\"],\"side\":\"RIGHT\"},\"type\":\"ConnectorPlacement.EquallySpacedRectSide\",\"uuid\":\"fe155757-f3d5-40d8-a583-dbbc24843437\"},{\"content\":{\"side\":\"TOP\"},\"type\":\"ConnectorPlacement.EquallySpacedRectSide\",\"uuid\":\"51bc4fd0-0675-45de-93bd-0dc8d94c5489\"}]},\"type\":\"ConnectorPlacement.EquallySpacedConnector\",\"uuid\":\"7eb8fdf8-dbe2-49f3-b9bd-384f85dcc997\"}],\"packageUris\":[\"http://schema.mathworks.com/mf0/Connector/R2020b\"],\"version\":\"1.0\"}"
  "XGCS49 L B201 " : Subsystem
      settings: PortSchema="{\"entries\":[{\"content\":{\"headerSize\":26,\"margin\":15,\"minimumSpacing\":25,\"sides\":[{\"content\":{},\"type\":\"ConnectorPlacement.EquallySpacedRectSide\",\"uuid\":\"ff8f3bf2-d6f6-4ecc-9677-a0e5f5ade440\"},{\"content\":{\"connectorIds\":[\"Out1\"],\"side\":\"RIGHT\"},\"type\":\"ConnectorPlacement.EquallySpacedRectSide\",\"uuid\":\"fe155757-f3d5-40d8-a583-dbbc24843437\"},{\"content\":{\"side\":\"TOP\"},\"type\":\"ConnectorPlacement.EquallySpacedRectSide\",\"uuid\":\"51bc4fd0-0675-45de-93bd-0dc8d94c5489\"}]},\"type\":\"ConnectorPlacement.EquallySpacedConnector\",\"uuid\":\"7eb8fdf8-dbe2-49f3-b9bd-384f85dcc997\"}],\"packageUris\":[\"http://schema.mathworks.com/mf0/Connector/R2020b\"],\"version\":\"1.0\"}"
  M18_rtu_data1 : Outport  PortName=M18_rtu_data
  M30_rtu_data1 : Outport  Port=2  PortName=M30_rtu_data
  XGCS49 0 1201_rtu_data1 : Outport  Port=3  PortName=XGCS49 0 1201_rtu_data
  XGCS 89 01201 _rtu_data1 : Outport  Port=4  PortName=XGCS 89 01201 _rtu_data
  XGCS49 0 B201 _rtu_data1 : Outport  Port=5  PortName=XGCS49 0 B201 _rtu_data
  XGCS49 L B201 _rtu_data1 : Outport  Port=6  PortName=XGCS49 L B201 _rtu_data
  wires:
  "XGCS 89 01201 "/1(XGCS 89 01201 _rtu_data) -> XGCS 89 01201 _rtu_data1/1
  "XGCS49 L B201 "/1(XGCS49 L B201 _rtu_data) -> XGCS49 L B201 _rtu_data1/1
  "XGCS49 0 B201 "/1(XGCS49 0 B201 _rtu_data) -> XGCS49 0 B201 _rtu_data1/1
  M18/1(M18_rtu_data) -> M18_rtu_data1/1
  M30/1(M30_rtu_data) -> M30_rtu_data1/1
  "XGCS49 0 1201 "/1(XGCS49 0 1201_rtu_data) -> XGCS49 0 1201_rtu_data1/1

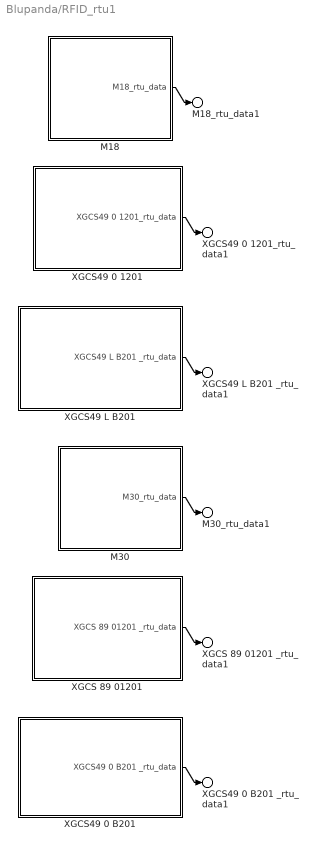
== system Blupanda/RFID_rtu1 ==
  M18 : Subsystem
      settings: PortSchema="{\"entries\":[{\"content\":{\"headerSize\":26,\"margin\":15,\"minimumSpacing\":25,\"sides\":[{\"content\":{},\"type\":\"ConnectorPlacement.EquallySpacedRectSide\",\"uuid\":\"ff8f3bf2-d6f6-4ecc-9677-a0e5f5ade440\"},{\"content\":{\"connectorIds\":[\"Out1\"],\"side\":\"RIGHT\"},\"type\":\"ConnectorPlacement.EquallySpacedRectSide\",\"uuid\":\"fe155757-f3d5-40d8-a583-dbbc24843437\"},{\"content\":{\"side\":\"TOP\"},\"type\":\"ConnectorPlacement.EquallySpacedRectSide\",\"uuid\":\"51bc4fd0-0675-45de-93bd-0dc8d94c5489\"}]},\"type\":\"ConnectorPlacement.EquallySpacedConnector\",\"uuid\":\"7eb8fdf8-dbe2-49f3-b9bd-384f85dcc997\"}],\"packageUris\":[\"http://schema.mathworks.com/mf0/Connector/R2020b\"],\"version\":\"1.0\"}"
  M30 : Subsystem
      settings: PortSchema="{\"entries\":[{\"content\":{\"headerSize\":26,\"margin\":15,\"minimumSpacing\":25,\"sides\":[{\"content\":{},\"type\":\"ConnectorPlacement.EquallySpacedRectSide\",\"uuid\":\"ff8f3bf2-d6f6-4ecc-9677-a0e5f5ade440\"},{\"content\":{\"connectorIds\":[\"Out1\"],\"side\":\"RIGHT\"},\"type\":\"ConnectorPlacement.EquallySpacedRectSide\",\"uuid\":\"fe155757-f3d5-40d8-a583-dbbc24843437\"},{\"content\":{\"side\":\"TOP\"},\"type\":\"ConnectorPlacement.EquallySpacedRectSide\",\"uuid\":\"51bc4fd0-0675-45de-93bd-0dc8d94c5489\"}]},\"type\":\"ConnectorPlacement.EquallySpacedConnector\",\"uuid\":\"7eb8fdf8-dbe2-49f3-b9bd-384f85dcc997\"}],\"packageUris\":[\"http://schema.mathworks.com/mf0/Connector/R2020b\"],\"version\":\"1.0\"}"
  "XGCS 89 01201 " : Subsystem
      settings: PortSchema="{\"entries\":[{\"content\":{\"headerSize\":26,\"margin\":15,\"minimumSpacing\":25,\"sides\":[{\"content\":{},\"type\":\"ConnectorPlacement.EquallySpacedRectSide\",\"uuid\":\"ff8f3bf2-d6f6-4ecc-9677-a0e5f5ade440\"},{\"content\":{\"connectorIds\":[\"Out1\"],\"side\":\"RIGHT\"},\"type\":\"ConnectorPlacement.EquallySpacedRectSide\",\"uuid\":\"fe155757-f3d5-40d8-a583-dbbc24843437\"},{\"content\":{\"side\":\"TOP\"},\"type\":\"ConnectorPlacement.EquallySpacedRectSide\",\"uuid\":\"51bc4fd0-0675-45de-93bd-0dc8d94c5489\"}]},\"type\":\"ConnectorPlacement.EquallySpacedConnector\",\"uuid\":\"7eb8fdf8-dbe2-49f3-b9bd-384f85dcc997\"}],\"packageUris\":[\"http://schema.mathworks.com/mf0/Connector/R2020b\"],\"version\":\"1.0\"}"
  "XGCS49 0 1201 " : Subsystem
      settings: PortSchema="{\"entries\":[{\"content\":{\"headerSize\":26,\"margin\":15,\"minimumSpacing\":25,\"sides\":[{\"content\":{},\"type\":\"ConnectorPlacement.EquallySpacedRectSide\",\"uuid\":\"ff8f3bf2-d6f6-4ecc-9677-a0e5f5ade440\"},{\"content\":{\"connectorIds\":[\"Out1\"],\"side\":\"RIGHT\"},\"type\":\"ConnectorPlacement.EquallySpacedRectSide\",\"uuid\":\"fe155757-f3d5-40d8-a583-dbbc24843437\"},{\"content\":{\"side\":\"TOP\"},\"type\":\"ConnectorPlacement.EquallySpacedRectSide\",\"uuid\":\"51bc4fd0-0675-45de-93bd-0dc8d94c5489\"}]},\"type\":\"ConnectorPlacement.EquallySpacedConnector\",\"uuid\":\"7eb8fdf8-dbe2-49f3-b9bd-384f85dcc997\"}],\"packageUris\":[\"http://schema.mathworks.com/mf0/Connector/R2020b\"],\"version\":\"1.0\"}"
  "XGCS49 0 B201 " : Subsystem
      settings: PortSchema="{\"entries\":[{\"content\":{\"headerSize\":26,\"margin\":15,\"minimumSpacing\":25,\"sides\":[{\"content\":{},\"type\":\"ConnectorPlacement.EquallySpacedRectSide\",\"uuid\":\"ff8f3bf2-d6f6-4ecc-9677-a0e5f5ade440\"},{\"content\":{\"connectorIds\":[\"Out1\"],\"side\":\"RIGHT\"},\"type\":\"ConnectorPlacement.EquallySpacedRectSide\",\"uuid\":\"fe155757-f3d5-40d8-a583-dbbc24843437\"},{\"content\":{\"side\":\"TOP\"},\"type\":\"ConnectorPlacement.EquallySpacedRectSide\",\"uuid\":\"51bc4fd0-0675-45de-93bd-0dc8d94c5489\"}]},\"type\":\"ConnectorPlacement.EquallySpacedConnector\",\"uuid\":\"7eb8fdf8-dbe2-49f3-b9bd-384f85dcc997\"}],\"packageUris\":[\"http://schema.mathworks.com/mf0/Connector/R2020b\"],\"version\":\"1.0\"}"
  "XGCS49 L B201 " : Subsystem
      settings: PortSchema="{\"entries\":[{\"content\":{\"headerSize\":26,\"margin\":15,\"minimumSpacing\":25,\"sides\":[{\"content\":{},\"type\":\"ConnectorPlacement.EquallySpacedRectSide\",\"uuid\":\"ff8f3bf2-d6f6-4ecc-9677-a0e5f5ade440\"},{\"content\":{\"connectorIds\":[\"Out1\"],\"side\":\"RIGHT\"},\"type\":\"ConnectorPlacement.EquallySpacedRectSide\",\"uuid\":\"fe155757-f3d5-40d8-a583-dbbc24843437\"},{\"content\":{\"side\":\"TOP\"},\"type\":\"ConnectorPlacement.EquallySpacedRectSide\",\"uuid\":\"51bc4fd0-0675-45de-93bd-0dc8d94c5489\"}]},\"type\":\"ConnectorPlacement.EquallySpacedConnector\",\"uuid\":\"7eb8fdf8-dbe2-49f3-b9bd-384f85dcc997\"}],\"packageUris\":[\"http://schema.mathworks.com/mf0/Connector/R2020b\"],\"version\":\"1.0\"}"
  M18_rtu_data1 : Outport  PortName=M18_rtu_data
  M30_rtu_data1 : Outport  Port=2  PortName=M30_rtu_data
  XGCS49 0 1201_rtu_data1 : Outport  Port=3  PortName=XGCS49 0 1201_rtu_data
  XGCS 89 01201 _rtu_data1 : Outport  Port=4  PortName=XGCS 89 01201 _rtu_data
  XGCS49 0 B201 _rtu_data1 : Outport  Port=5  PortName=XGCS49 0 B201 _rtu_data
  XGCS49 L B201 _rtu_data1 : Outport  Port=6  PortName=XGCS49 L B201 _rtu_data
  wires:
  "XGCS 89 01201 "/1(XGCS 89 01201 _rtu_data) -> XGCS 89 01201 _rtu_data1/1
  "XGCS49 L B201 "/1(XGCS49 L B201 _rtu_data) -> XGCS49 L B201 _rtu_data1/1
  "XGCS49 0 B201 "/1(XGCS49 0 B201 _rtu_data) -> XGCS49 0 B201 _rtu_data1/1
  M18/1(M18_rtu_data) -> M18_rtu_data1/1
  M30/1(M30_rtu_data) -> M30_rtu_data1/1
  "XGCS49 0 1201 "/1(XGCS49 0 1201_rtu_data) -> XGCS49 0 1201_rtu_data1/1

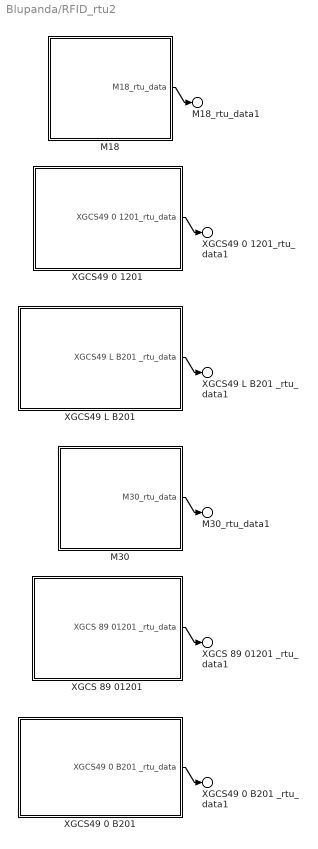
== system Blupanda/RFID_rtu2 ==
  M18 : Subsystem
      settings: PortSchema="{\"entries\":[{\"content\":{\"headerSize\":26,\"margin\":15,\"minimumSpacing\":25,\"sides\":[{\"content\":{},\"type\":\"ConnectorPlacement.EquallySpacedRectSide\",\"uuid\":\"ff8f3bf2-d6f6-4ecc-9677-a0e5f5ade440\"},{\"content\":{\"connectorIds\":[\"Out1\"],\"side\":\"RIGHT\"},\"type\":\"ConnectorPlacement.EquallySpacedRectSide\",\"uuid\":\"fe155757-f3d5-40d8-a583-dbbc24843437\"},{\"content\":{\"side\":\"TOP\"},\"type\":\"ConnectorPlacement.EquallySpacedRectSide\",\"uuid\":\"51bc4fd0-0675-45de-93bd-0dc8d94c5489\"}]},\"type\":\"ConnectorPlacement.EquallySpacedConnector\",\"uuid\":\"7eb8fdf8-dbe2-49f3-b9bd-384f85dcc997\"}],\"packageUris\":[\"http://schema.mathworks.com/mf0/Connector/R2020b\"],\"version\":\"1.0\"}"
  M30 : Subsystem
      settings: PortSchema="{\"entries\":[{\"content\":{\"headerSize\":26,\"margin\":15,\"minimumSpacing\":25,\"sides\":[{\"content\":{},\"type\":\"ConnectorPlacement.EquallySpacedRectSide\",\"uuid\":\"ff8f3bf2-d6f6-4ecc-9677-a0e5f5ade440\"},{\"content\":{\"connectorIds\":[\"Out1\"],\"side\":\"RIGHT\"},\"type\":\"ConnectorPlacement.EquallySpacedRectSide\",\"uuid\":\"fe155757-f3d5-40d8-a583-dbbc24843437\"},{\"content\":{\"side\":\"TOP\"},\"type\":\"ConnectorPlacement.EquallySpacedRectSide\",\"uuid\":\"51bc4fd0-0675-45de-93bd-0dc8d94c5489\"}]},\"type\":\"ConnectorPlacement.EquallySpacedConnector\",\"uuid\":\"7eb8fdf8-dbe2-49f3-b9bd-384f85dcc997\"}],\"packageUris\":[\"http://schema.mathworks.com/mf0/Connector/R2020b\"],\"version\":\"1.0\"}"
  "XGCS 89 01201 " : Subsystem
      settings: PortSchema="{\"entries\":[{\"content\":{\"headerSize\":26,\"margin\":15,\"minimumSpacing\":25,\"sides\":[{\"content\":{},\"type\":\"ConnectorPlacement.EquallySpacedRectSide\",\"uuid\":\"ff8f3bf2-d6f6-4ecc-9677-a0e5f5ade440\"},{\"content\":{\"connectorIds\":[\"Out1\"],\"side\":\"RIGHT\"},\"type\":\"ConnectorPlacement.EquallySpacedRectSide\",\"uuid\":\"fe155757-f3d5-40d8-a583-dbbc24843437\"},{\"content\":{\"side\":\"TOP\"},\"type\":\"ConnectorPlacement.EquallySpacedRectSide\",\"uuid\":\"51bc4fd0-0675-45de-93bd-0dc8d94c5489\"}]},\"type\":\"ConnectorPlacement.EquallySpacedConnector\",\"uuid\":\"7eb8fdf8-dbe2-49f3-b9bd-384f85dcc997\"}],\"packageUris\":[\"http://schema.mathworks.com/mf0/Connector/R2020b\"],\"version\":\"1.0\"}"
  "XGCS49 0 1201 " : Subsystem
      settings: PortSchema="{\"entries\":[{\"content\":{\"headerSize\":26,\"margin\":15,\"minimumSpacing\":25,\"sides\":[{\"content\":{},\"type\":\"ConnectorPlacement.EquallySpacedRectSide\",\"uuid\":\"ff8f3bf2-d6f6-4ecc-9677-a0e5f5ade440\"},{\"content\":{\"connectorIds\":[\"Out1\"],\"side\":\"RIGHT\"},\"type\":\"ConnectorPlacement.EquallySpacedRectSide\",\"uuid\":\"fe155757-f3d5-40d8-a583-dbbc24843437\"},{\"content\":{\"side\":\"TOP\"},\"type\":\"ConnectorPlacement.EquallySpacedRectSide\",\"uuid\":\"51bc4fd0-0675-45de-93bd-0dc8d94c5489\"}]},\"type\":\"ConnectorPlacement.EquallySpacedConnector\",\"uuid\":\"7eb8fdf8-dbe2-49f3-b9bd-384f85dcc997\"}],\"packageUris\":[\"http://schema.mathworks.com/mf0/Connector/R2020b\"],\"version\":\"1.0\"}"
  "XGCS49 0 B201 " : Subsystem
      settings: PortSchema="{\"entries\":[{\"content\":{\"headerSize\":26,\"margin\":15,\"minimumSpacing\":25,\"sides\":[{\"content\":{},\"type\":\"ConnectorPlacement.EquallySpacedRectSide\",\"uuid\":\"ff8f3bf2-d6f6-4ecc-9677-a0e5f5ade440\"},{\"content\":{\"connectorIds\":[\"Out1\"],\"side\":\"RIGHT\"},\"type\":\"ConnectorPlacement.EquallySpacedRectSide\",\"uuid\":\"fe155757-f3d5-40d8-a583-dbbc24843437\"},{\"content\":{\"side\":\"TOP\"},\"type\":\"ConnectorPlacement.EquallySpacedRectSide\",\"uuid\":\"51bc4fd0-0675-45de-93bd-0dc8d94c5489\"}]},\"type\":\"ConnectorPlacement.EquallySpacedConnector\",\"uuid\":\"7eb8fdf8-dbe2-49f3-b9bd-384f85dcc997\"}],\"packageUris\":[\"http://schema.mathworks.com/mf0/Connector/R2020b\"],\"version\":\"1.0\"}"
  "XGCS49 L B201 " : Subsystem
      settings: PortSchema="{\"entries\":[{\"content\":{\"headerSize\":26,\"margin\":15,\"minimumSpacing\":25,\"sides\":[{\"content\":{},\"type\":\"ConnectorPlacement.EquallySpacedRectSide\",\"uuid\":\"ff8f3bf2-d6f6-4ecc-9677-a0e5f5ade440\"},{\"content\":{\"connectorIds\":[\"Out1\"],\"side\":\"RIGHT\"},\"type\":\"ConnectorPlacement.EquallySpacedRectSide\",\"uuid\":\"fe155757-f3d5-40d8-a583-dbbc24843437\"},{\"content\":{\"side\":\"TOP\"},\"type\":\"ConnectorPlacement.EquallySpacedRectSide\",\"uuid\":\"51bc4fd0-0675-45de-93bd-0dc8d94c5489\"}]},\"type\":\"ConnectorPlacement.EquallySpacedConnector\",\"uuid\":\"7eb8fdf8-dbe2-49f3-b9bd-384f85dcc997\"}],\"packageUris\":[\"http://schema.mathworks.com/mf0/Connector/R2020b\"],\"version\":\"1.0\"}"
  M18_rtu_data1 : Outport  PortName=M18_rtu_data
  M30_rtu_data1 : Outport  Port=2  PortName=M30_rtu_data
  XGCS49 0 1201_rtu_data1 : Outport  Port=3  PortName=XGCS49 0 1201_rtu_data
  XGCS 89 01201 _rtu_data1 : Outport  Port=4  PortName=XGCS 89 01201 _rtu_data
  XGCS49 0 B201 _rtu_data1 : Outport  Port=5  PortName=XGCS49 0 B201 _rtu_data
  XGCS49 L B201 _rtu_data1 : Outport  Port=6  PortName=XGCS49 L B201 _rtu_data
  wires:
  "XGCS 89 01201 "/1(XGCS 89 01201 _rtu_data) -> XGCS 89 01201 _rtu_data1/1
  "XGCS49 L B201 "/1(XGCS49 L B201 _rtu_data) -> XGCS49 L B201 _rtu_data1/1
  "XGCS49 0 B201 "/1(XGCS49 0 B201 _rtu_data) -> XGCS49 0 B201 _rtu_data1/1
  M18/1(M18_rtu_data) -> M18_rtu_data1/1
  M30/1(M30_rtu_data) -> M30_rtu_data1/1
  "XGCS49 0 1201 "/1(XGCS49 0 1201_rtu_data) -> XGCS49 0 1201_rtu_data1/1

== system Blupanda/TCSESU051F0 ==
  Bus Element In3 : Inport  PortName=IOLink_master_Profinet_serial_data_EthernetIP
  Bus Element In1 : Inport  Port=2  PortName=XGSZ 84 EIP _serial_data_ethernet_2_network
  Bus Element In2 : Inport  Port=3  PortName=XGCS 850C 201_Ethernetp_Data_2_swtich
  Bus Element Out1 : Outport  PortName=ethernet ip data

== system Blupanda/XGSZ 84 EIP  ==
  Bus Element In1 : Inport  PortName=M18_rtu_data_2_ethernet_box
  Bus Element In2 : Inport  Port=2  PortName=M30_rtu_data_2_ethernet_box
  Bus Element In3 : Inport  Port=3  PortName=XGCS49 0 1201_rtu_data_2_ethernet_box
  Bus Element In4 : Inport  Port=4  PortName=XGCS49 0 B201 _rtu_data_2_ethernet_box
  Bus Element In5 : Inport  Port=5  PortName=XGCS49 L B201 _rtu_data_2_ethernet_box
  Bus Element In6 : Inport  Port=6  PortName=XGCS 89 01201 _rtu_data_2_ethernet_box
  Bus Element Out1 : Outport  PortName=XGSZ 84 EIP _serial_data_ethernet

== system Blupanda/XGSZ 84 ETH  ==
  Bus Element In1 : Inport  PortName=M18_rtu_data_2_modbus_ box
  Bus Element In2 : Inport  Port=2  PortName=M30_rtu_data_2_modbus_box
  Bus Element In3 : Inport  Port=3  PortName=XGCS49 0 1201_rtu_data_2_modbus_box
  Bus Element In4 : Inport  Port=4  PortName=XGCS49 0 B201 _rtu_data_2_modbus_box
  Bus Element In5 : Inport  Port=5  PortName=XGCS49 L B201 _rtu_data_2_modbus_box
  Bus Element In6 : Inport  Port=6  PortName=XGCS 89 01201 _rtu_data_2_modbus_box
  Bus Element Out1 : Outport  PortName=XGSZ84 ETH _serial_data_Mobdus

== system Blupanda/XGSZ84 PNT  ==
  Bus Element In1 : Inport  PortName=""
  Bus Element In2 : Inport  Port=2  PortName=M30_rtu_data_2_profinet_box
  Bus Element In3 : Inport  Port=3  PortName=XGCS49 0 1201_rtu_data_2_profinet_box
  Bus Element In4 : Inport  Port=4  PortName=XGCS49 0 B201 _rtu_data_2_profinet_box
  Bus Element In5 : Inport  Port=5  PortName=XGCS49 L B201 _rtu_data_2_profinet_box
  Bus Element In6 : Inport  Port=6  PortName=XGCS 89 01201 _rtu_data_2_profinet_box
  Bus Element Out1 : Outport  PortName="XGSZ84 PNT  _serial_data_Profinet"

== system Blupanda/Control Module/CANJ Interface ==
  Bus Element In1 : Inport  PortName=CANJ_Sensor_fieldbus
  Bus Element Out1 : Outport  PortName=CANJ_Interface_Data

== system Blupanda/Control Module/Ethernet Interface ==
  Bus Element In1 : Inport  PortName=Ethernetip_Sensor_fieldbus
  Bus Element Out1 : Outport  PortName=Ethernet_Interface_Data

== system Blupanda/Control Module/IO Module ==
  Bus Element In1 : Inport  PortName=Descrete/Analog Input
  Bus Element Out1 : Outport  PortName=Descrete/Analog Data

== system Blupanda/Control Module/Modbus IIntereface ==
  Bus Element In1 : Inport  PortName=Modbus_Sensor_fieldbus
  Bus Element Out1 : Outport  PortName=Modbus_Intereface_Data

== system Blupanda/Control Module/PLC ==
  Bus Element In6 : Inport  PortName=Descrete/Analog Data
  Bus Element In5 : Inport  Port=2  PortName=CANJ_Interface_Data
  Bus Element In4 : Inport  Port=3  PortName=PLC_Programmation
  Bus Element In1 : Inport  Port=4  PortName=Profinet_Interface_Data
  Bus Element In2 : Inport  Port=5  PortName=Ethernet_Interface_Data
  Bus Element In3 : Inport  Port=6  PortName=Modbus_Intereface_Data
  Bus Element Out1 : Outport  PortName=Process_Parameters_HMI

== system Blupanda/Control Module/Profinet Interface ==
  Bus Element In1 : Inport  PortName=Profinet_Sensor_fieldbus
  Bus Element Out1 : Outport  PortName=Profinet_Interface_Data

== system Blupanda/RFID_CANJ/XGCS460B201 ==
  Bus Element Out1 : Outport  PortName=XGCS460B201_CANJ_Data

== system Blupanda/RFID_EthernetIP/XGCS 850C 201  ==
  Bus Element Out1 : Outport  PortName=XGCS 850C 201_Ethernetp_Data

== system Blupanda/RFID_IO_Link/M18 ==
  Bus Element Out1 : Outport  PortName=M18_IOLink_data

== system Blupanda/RFID_IO_Link/M30 ==
  Bus Element Out1 : Outport  PortName=M30_IOLink_data

== system Blupanda/RFID_IO_Link/XGCS 49 01201 ==
  Bus Element Out1 : Outport  PortName=XGCS 49 01201_IOLink_data

== system Blupanda/RFID_IO_Link/XGCS 89 01201 ==
  Bus Element Out1 : Outport  PortName=XGCS 89 01201_IOLimk_data

== system Blupanda/RFID_IO_Link1/M18 ==
  Bus Element Out1 : Outport  PortName=M18_IOLink_data

== system Blupanda/RFID_IO_Link1/M30 ==
  Bus Element Out1 : Outport  PortName=M30_IOLink_data

== system Blupanda/RFID_IO_Link1/XGCS 49 01201 ==
  Bus Element Out1 : Outport  PortName=XGCS 49 01201_IOLink_data

== system Blupanda/RFID_IO_Link1/XGCS 89 01201 ==
  Bus Element Out1 : Outport  PortName=XGCS 89 01201_IOLimk_data

== system Blupanda/RFID_Modbus/XGCS 850C 201 ==
  Bus Element Out1 : Outport  PortName=XGCS 850C 201_ModusTCp_Data

== system Blupanda/RFID_PNP/XGCS49 1 B201  ==
  Bus Element In2 : Inport  PortName=InBus1
  Bus Element In1 : Inport  Port=2  PortName=InBus
  Bus Element Out1 : Outport  PortName=XGCS49 1 B201_PNP_Data

== system Blupanda/RFID_Profinet/XGCS 850C 201  ==
  Bus Element Out1 : Outport  PortName=XGCS 850C 201_Profinet_Data

== system Blupanda/RFID_rtu/M18 ==
  Bus Element Out1 : Outport  PortName=M18_rtu_data

== system Blupanda/RFID_rtu/M30 ==
  Bus Element Out1 : Outport  PortName=M30_rtu_data

== system Blupanda/RFID_rtu/XGCS 89 01201  ==
  Bus Element Out1 : Outport  PortName=XGCS 89 01201 _rtu_data

== system Blupanda/RFID_rtu/XGCS49 0 1201  ==
  Bus Element Out1 : Outport  PortName=XGCS49 0 1201_rtu_data

== system Blupanda/RFID_rtu/XGCS49 0 B201  ==
  Bus Element Out1 : Outport  PortName=XGCS49 0 B201 _rtu_data

== system Blupanda/RFID_rtu/XGCS49 L B201  ==
  Bus Element Out1 : Outport  PortName=XGCS49 L B201 _rtu_data

== system Blupanda/RFID_rtu1/M18 ==
  Bus Element Out1 : Outport  PortName=M18_rtu_data

== system Blupanda/RFID_rtu1/M30 ==
  Bus Element Out1 : Outport  PortName=M30_rtu_data

== system Blupanda/RFID_rtu1/XGCS 89 01201  ==
  Bus Element Out1 : Outport  PortName=XGCS 89 01201 _rtu_data

== system Blupanda/RFID_rtu1/XGCS49 0 1201  ==
  Bus Element Out1 : Outport  PortName=XGCS49 0 1201_rtu_data

== system Blupanda/RFID_rtu1/XGCS49 0 B201  ==
  Bus Element Out1 : Outport  PortName=XGCS49 0 B201 _rtu_data

== system Blupanda/RFID_rtu1/XGCS49 L B201  ==
  Bus Element Out1 : Outport  PortName=XGCS49 L B201 _rtu_data

== system Blupanda/RFID_rtu2/M18 ==
  Bus Element Out1 : Outport  PortName=M18_rtu_data

== system Blupanda/RFID_rtu2/M30 ==
  Bus Element Out1 : Outport  PortName=M30_rtu_data

== system Blupanda/RFID_rtu2/XGCS 89 01201  ==
  Bus Element Out1 : Outport  PortName=XGCS 89 01201 _rtu_data

== system Blupanda/RFID_rtu2/XGCS49 0 1201  ==
  Bus Element Out1 : Outport  PortName=XGCS49 0 1201_rtu_data

== system Blupanda/RFID_rtu2/XGCS49 0 B201  ==
  Bus Element Out1 : Outport  PortName=XGCS49 0 B201 _rtu_data

== system Blupanda/RFID_rtu2/XGCS49 L B201  ==
  Bus Element Out1 : Outport  PortName=XGCS49 L B201 _rtu_data
